simulink library "NG_CHP_lib"  (Simulink 8.1)
settings: Solver=ode45  StartTime=0.0  StopTime=10.0  RelTol=1e-3
undefined symbols (not defined in the file): fdesignblkfcn, gcbh, ph, SIM_HIL, Ts
libraries: simulink x23, rtio_opalrt_common x21, simulink_extras x6, rteventslib x4, CHP_Model_lib x1, NG_Genset_lib x1, rtio_generic_modbus x1
(part 2 of 2)

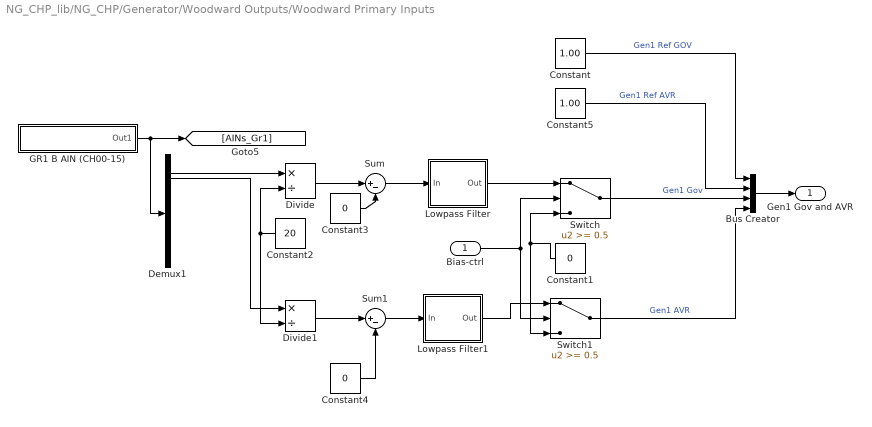
== system NG_CHP_lib/NG_CHP/Generator/Woodward Outputs/Woodward Primary Inputs ==
  Bias-ctrl : Inport
  Bus Creator : BusCreator
  Constant : Constant  Value=1.00
  Constant1 : Constant  Value=0
  Constant2 : Constant  Value=20
  Constant3 : Constant  Value=0
  Constant4 : Constant  Value=0
  Constant5 : Constant  Value=1.00
  Demux1 : Demux  Outputs=16
  Divide : Product  Inputs=*/
  Divide1 : Product  Inputs=*/
  GR1 B AIN (CH00-15) : Subsystem
  Lowpass Filter : Subsystem  DialogController=fdesignblkfcn  DialogControllerArgs=DataTag1  InitFcn=fdesignblkfcn(gcbh, {'InitFcn'});  mask(Lowpass Filter){}
      mask help: Design a lowpass filter
      settings: CopyFcn=fdesignblkfcn(gcbh, {'CopyFcn'});
      mask Help: helpview(mapfilelocation('dsp'), 'dsplowpassfilter');
      mask Display: disp('Lowpass')
  Lowpass Filter1 : Subsystem  DialogController=fdesignblkfcn  DialogControllerArgs=DataTag3  InitFcn=fdesignblkfcn(gcbh, {'InitFcn'});  mask(Lowpass Filter){}
      mask help: Design a lowpass filter
      settings: CopyFcn=fdesignblkfcn(gcbh, {'CopyFcn'});
      mask Help: helpview(mapfilelocation('dsp'), 'dsplowpassfilter');
      mask Display: disp('Lowpass')
  Sum : Sum  Inputs=|+-
  Sum1 : Sum  Inputs=|+-
  Switch : Switch  Threshold=0.5
  Switch1 : Switch  Threshold=0.5
  Gen1 Gov and AVR : Outport
  wires:
  GR1 B AIN (CH00-15)/1(Out1) -> [AINs_Gr1], Demux1/1
  Demux1/1 -> Divide/1
  Demux1/2 -> Divide1/1
  Constant2/1 -> Divide1/2, Divide/2
  Divide/1 -> Sum/1
  Divide1/1 -> Sum1/1
  Constant3/1 -> Sum/2
  Constant4/1 -> Sum1/2
  Sum/1 -> Lowpass Filter/1(In)
  Switch/1 -> Bus Creator/3  "Gen1 Gov"
  Switch1/1 -> Bus Creator/4  "Gen1 AVR"
  Sum1/1 -> Lowpass Filter1/1(In)
  Constant1/1 -> Switch/3, Switch1/3
  Bias-ctrl/1 -> Switch/2, Switch1/2
  Lowpass Filter/1(Out) -> Switch/1
  Lowpass Filter1/1(Out) -> Switch1/1
  Constant5/1 -> Bus Creator/2  "Gen1 Ref AVR"
  Constant/1 -> Bus Creator/1  "Gen1 Ref GOV"
  Bus Creator/1 -> Gen1 Gov and AVR/1

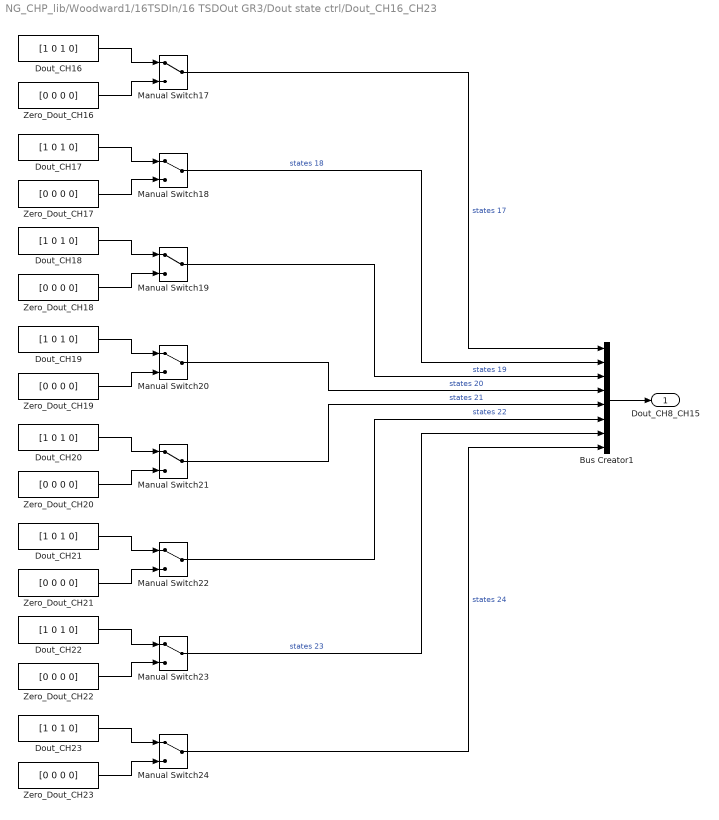
== system NG_CHP_lib/Woodward1/16TSDIn/16 TSDOut GR3/Dout state ctrl/Dout_CH16_CH23 ==
  Bus Creator1 : BusCreator  Inputs=8
  Dout_CH{16..23} (8 alike) : Constant  Value=[1 0 1 0]
  Manual Switch{17..24} (8 alike) : ManualSwitch
  Zero_Dout_CH{16..23} (8 alike) : Constant  Value=[0 0 0 0]
  Dout_CH8_CH15 : Outport
  wires:
  Manual Switch24/1 -> Bus Creator1/8  "states 24"
  Manual Switch23/1 -> Bus Creator1/7  "states 23"
  Manual Switch22/1 -> Bus Creator1/6  "states 22"
  Manual Switch21/1 -> Bus Creator1/5  "states 21"
  Manual Switch20/1 -> Bus Creator1/4  "states 20"
  Manual Switch19/1 -> Bus Creator1/3  "states 19"
  Manual Switch18/1 -> Bus Creator1/2  "states 18"
  Manual Switch17/1 -> Bus Creator1/1  "states 17"
  Zero_Dout_CH23/1 -> Manual Switch24/2
  Dout_CH23/1 -> Manual Switch24/1
  Zero_Dout_CH22/1 -> Manual Switch23/2
  Dout_CH22/1 -> Manual Switch23/1
  Zero_Dout_CH21/1 -> Manual Switch22/2
  Dout_CH21/1 -> Manual Switch22/1
  Zero_Dout_CH20/1 -> Manual Switch21/2
  Dout_CH20/1 -> Manual Switch21/1
  Zero_Dout_CH19/1 -> Manual Switch20/2
  Dout_CH19/1 -> Manual Switch20/1
  Zero_Dout_CH18/1 -> Manual Switch19/2
  Dout_CH18/1 -> Manual Switch19/1
  Zero_Dout_CH17/1 -> Manual Switch18/2
  Dout_CH17/1 -> Manual Switch18/1
  Zero_Dout_CH16/1 -> Manual Switch17/2
  Dout_CH16/1 -> Manual Switch17/1
  Bus Creator1/1 -> Dout_CH8_CH15/1

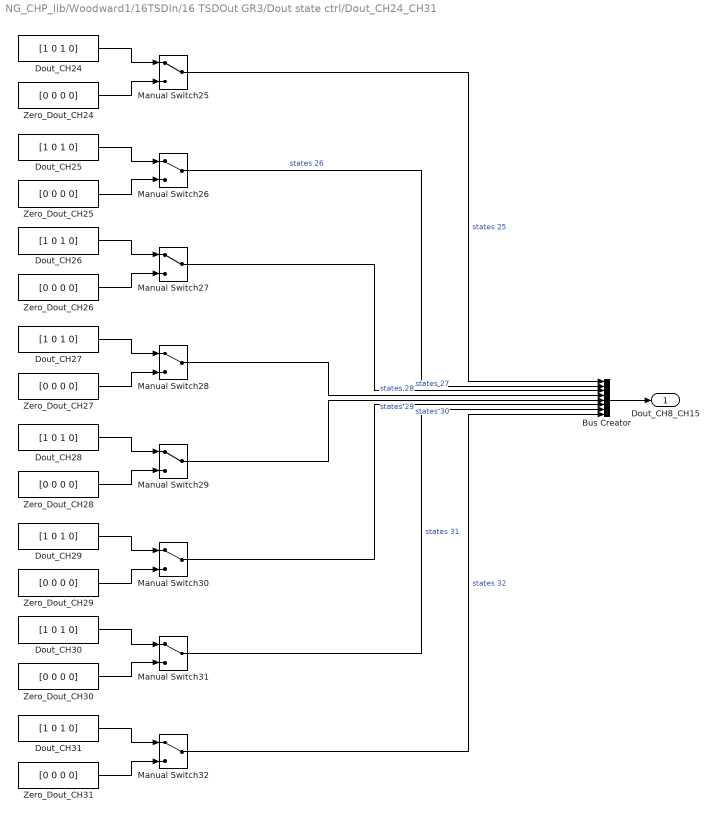
== system NG_CHP_lib/Woodward1/16TSDIn/16 TSDOut GR3/Dout state ctrl/Dout_CH24_CH31 ==
  Bus Creator : BusCreator  Inputs=8
  Dout_CH{24..31} (8 alike) : Constant  Value=[1 0 1 0]
  Manual Switch{25..32} (8 alike) : ManualSwitch
  Zero_Dout_CH{24..31} (8 alike) : Constant  Value=[0 0 0 0]
  Dout_CH8_CH15 : Outport
  wires:
  Bus Creator/1 -> Dout_CH8_CH15/1
  Dout_CH24/1 -> Manual Switch25/1
  Zero_Dout_CH24/1 -> Manual Switch25/2
  Dout_CH25/1 -> Manual Switch26/1
  Zero_Dout_CH25/1 -> Manual Switch26/2
  Dout_CH26/1 -> Manual Switch27/1
  Zero_Dout_CH26/1 -> Manual Switch27/2
  Dout_CH27/1 -> Manual Switch28/1
  Zero_Dout_CH27/1 -> Manual Switch28/2
  Dout_CH28/1 -> Manual Switch29/1
  Zero_Dout_CH28/1 -> Manual Switch29/2
  Dout_CH29/1 -> Manual Switch30/1
  Zero_Dout_CH29/1 -> Manual Switch30/2
  Dout_CH30/1 -> Manual Switch31/1
  Zero_Dout_CH30/1 -> Manual Switch31/2
  Dout_CH31/1 -> Manual Switch32/1
  Zero_Dout_CH31/1 -> Manual Switch32/2
  Manual Switch25/1 -> Bus Creator/1  "states 25"
  Manual Switch26/1 -> Bus Creator/2  "states 26"
  Manual Switch27/1 -> Bus Creator/3  "states 27"
  Manual Switch28/1 -> Bus Creator/4  "states 28"
  Manual Switch29/1 -> Bus Creator/5  "states 29"
  Manual Switch30/1 -> Bus Creator/6  "states 30"
  Manual Switch31/1 -> Bus Creator/7  "states 31"
  Manual Switch32/1 -> Bus Creator/8  "states 32"

== system NG_CHP_lib/NG_CHP/Generator/Woodward Outputs/DIO - Gr3/Conditioning ==
  In1 : Inport
  Bus Creator : BusCreator  Inputs=8
  Demux : Demux  Outputs=8
  Out1 : Outport
  wires:
  Demux/1 -> Bus Creator/1  "Gen1_Starter"
  Demux/2 -> Bus Creator/2  "Gen1_Fuel"
  Demux/3 -> Bus Creator/3  "Gen1_Close_GCB"
  Demux/4 -> Bus Creator/4  "Gen1_Open_GCB"
  Demux/5 -> Bus Creator/5  "Gen1_Close_MCB"
  Demux/6 -> Bus Creator/6  "Gen1_Open_MCB"
  Demux/7 -> Bus Creator/7  "Gen1_Alarm_AB"
  Demux/8 -> Bus Creator/8  "Gen1_Alarm_CF"
  Bus Creator/1 -> Out1/1  "DI_CH00-07"
  In1/1 -> Demux/1

== system NG_CHP_lib/NG_CHP/Generator/Woodward Outputs/DIO - Gr3/Conditioning1 ==
  In1 : Inport
  Bus Creator : BusCreator  Inputs=8
  Demux : Demux  Outputs=8
  Out1 : Outport
  wires:
  In1/1 -> Demux/1
  Bus Creator/1 -> Out1/1  "DI_CH08-15"
  Demux/8 -> Bus Creator/8  "Gen2_Alarm_CF"
  Demux/7 -> Bus Creator/7  "Gen2_Alarm_AB"
  Demux/6 -> Bus Creator/6  "Gen2_Open_MCB"
  Demux/5 -> Bus Creator/5  "Gen2_Close_MCB"
  Demux/4 -> Bus Creator/4  "Gen2_Open_GCB"
  Demux/3 -> Bus Creator/3  "Gen2_Close_GCB"
  Demux/2 -> Bus Creator/2  "Gen2_Fuel"
  Demux/1 -> Bus Creator/1  "Gen2_Starter"

== system NG_CHP_lib/NG_CHP/Generator/Woodward Outputs/Woodward Primary Inputs/GR1 B AIN (CH00-15) ==
  AnalogIn : rtio_opalrt_common/AnalogIn  CtrlName='OpCtrl'  portNb=1  FcnNos=Slot 1 Module B Subsection 1  size=16  maxcount=-2  count=-2  numchan=-2  sampleTime=0
      settings: AttributesFormatString=%<CtrlName>
  AnalogIn1 : rtio_opalrt_common/AnalogIn  CtrlName='OpCtrl'  portNb=2  FcnNos=Slot 1 Module B Subsection 2  size=16  maxcount=-2  count=-2  numchan=-2  sampleTime=0
      settings: AttributesFormatString=%<CtrlName>
  Mux6 : Mux  Inputs=2
  Terminator2 : Terminator
  Terminator3 : Terminator
  Out1 : Outport
  wires:
  Mux6/1 -> Out1/1
  AnalogIn1/2 -> Terminator3/1
  AnalogIn/2 -> Terminator2/1
  AnalogIn1/1 -> Mux6/2
  AnalogIn/1 -> Mux6/1

== system NG_CHP_lib/NG_CHP/Generator/Woodward Outputs/Woodward Primary Inputs/Lowpass Filter ==
  In : Inport
  Generated Filter Block : DiscreteFir  Tag=BlockMethodSubSystem  Coefficients=[0.0069552863617617106 0.014587901014631248 -0.0057896483056441538 -0.056861876528372622 -0.059476680260783142 0.076118200884714562 0.29579154768342669 0.40638624201187618 0.29579154768342669 0.076118200884714562 -0.059476680260783142 -0.056861876528372622 -0.0057896483056441538 0.014587901014631248 0.0069552863617617106]  InputProcessing=Columns as channels (frame based)
  Out : Outport
  wires:
  In/1 -> Generated Filter Block/1
  Generated Filter Block/1 -> Out/1

== system NG_CHP_lib/NG_CHP/Generator/Woodward Outputs/Woodward Primary Inputs/Lowpass Filter1 ==
  In : Inport
  Generated Filter Block : DiscreteFir  Tag=BlockMethodSubSystem  Coefficients=[0.0069552863617617106 0.014587901014631248 -0.0057896483056441538 -0.056861876528372622 -0.059476680260783142 0.076118200884714562 0.29579154768342669 0.40638624201187618 0.29579154768342669 0.076118200884714562 -0.059476680260783142 -0.056861876528372622 -0.0057896483056441538 0.014587901014631248 0.0069552863617617106]  InputProcessing=Columns as channels (frame based)
  Out : Outport
  wires:
  In/1 -> Generated Filter Block/1
  Generated Filter Block/1 -> Out/1
